simulink model "Calculatrice_vierge"  (R2016b)
settings: Solver=VariableStepAuto  StartTime=0.0  StopTime=10.0  RelTol=1e-3
libraries: commutil2 x3
settings Model: Creator=rcostado  LastModifiedBy=rcostado

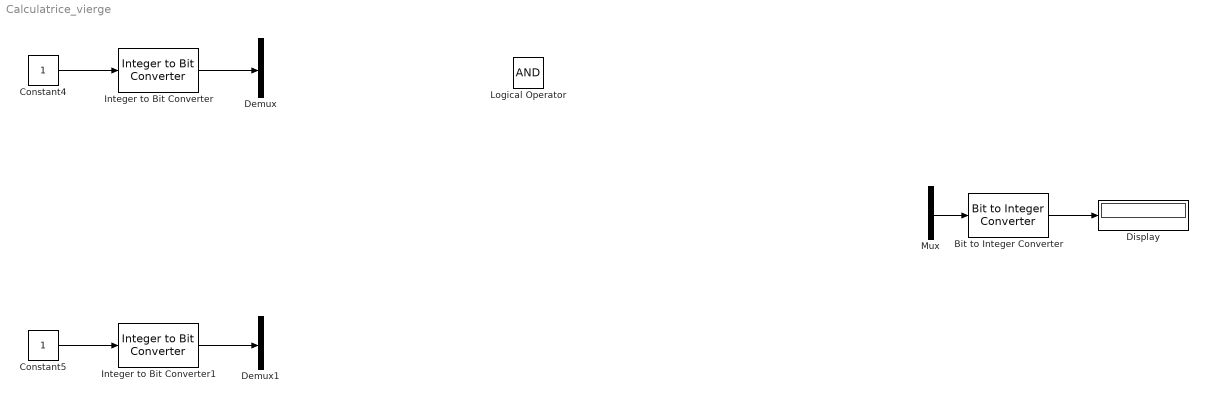
== system Calculatrice_vierge ==
  Bit to Integer Converter : commutil2/Bit to Integer Converter  nbits=4  bitOrder=MSB first  signedOutputValues=Unsigned  outDtype=Inherit via internal rule  outDtypeSigned=Inherit via internal rule
  Constant4 : Constant
  Constant5 : Constant
  Demux : Demux
  Demux1 : Demux
  Display : Display
  Integer to Bit Converter : commutil2/Integer to Bit Converter  nbits=4  signedInputValues=Unsigned  bitOrder=MSB first  outDtype=Inherit via internal rule
  Integer to Bit Converter1 : commutil2/Integer to Bit Converter  nbits=4  signedInputValues=Unsigned  bitOrder=MSB first  outDtype=Inherit via internal rule
  Logical Operator : Logic  AllPortsSameDT=off  OutDataTypeStr=boolean
  Mux : Mux
  wires:
  Mux/1 -> Bit to Integer Converter/1
  Bit to Integer Converter/1 -> Display/1
  Integer to Bit Converter1/1 -> Demux1/1
  Constant5/1 -> Integer to Bit Converter1/1
  Constant4/1 -> Integer to Bit Converter/1
  Integer to Bit Converter/1 -> Demux/1
